simulink model "MyPowerSupply_RTW"  (Simulink 7.5)
settings: Solver=ode1  SolverMode=SingleTasking  StartTime=0.0  StopTime=inf  FixedStep=0.0002  RelTol=1e-3
PreLoadFcn:
  | vehicle = 'Car'; if ~length(which('cmcmd')), cmenv; end
  | MyPowerSupply_RTW_bus
InitFcn:
  | vehicle = 'Car'; if ~length(which('cmcmd')), cmenv; end
  | MyPowerSupply_RTW_bus
libraries: simulink x3, CarMaker4SL x3
Description:
  | CarMaker Real-Time Target (generic)
settings Model: Creator=ml  LastModifiedBy=ml
settings DebuggingCC: SolverPrmCheckMsg=none
settings HardwareCC: TargetHWDeviceType=32-bit Generic  ProdEqTarget=off
settings RTWCC: SystemTargetFile=CarMaker.tlc  TemplateMakefile=CarMaker_unix.tmf  Description=CarMaker Real-Time Target (32-bit)  ProcessScript=CarMaker_make_rtw_hook
settings CodeAppCC: MaxIdLength=63
settings STFCustomTargetCC: ModelReferenceCompliant=off  GeneratePreprocessorConditionals=Disable all  SystemTargetFile=CarMaker.tlc
settings GRTTargetCC: ModelReferenceCompliant=off  ParMdlRefBuildCompliant=off  CompOptLevelCompliant=off  MatFileLogging=off  ExtModeMexFile=noextcomm
settings CustomProperty: DataType=string  Value=..
settings EnumStrPairs: String=Car

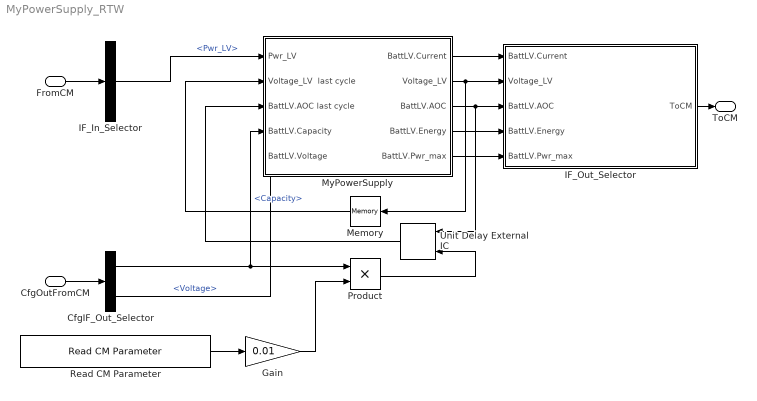
== system MyPowerSupply_RTW ==
  FromCM : Inport  UseBusObject=on
      settings: BusObject=cmPTPowerSupplyIn
  CfgOutFromCM : Inport  Port=2  UseBusObject=on
      settings: BusObject=cmPTPowerSupplyCfgOut
  CfgIF_Out_Selector : BusSelector  OutputSignals=BattLV.Capacity,BattLV.Voltage
  Gain : Gain  Gain=0.01  ParameterDataType=sfix(16)  ParameterScaling=2^0  OutDataType=sfix(16)  OutScaling=2^0
  IF_In_Selector : BusSelector  OutputSignals=Pwr_LV
  IF_Out_Selector : Subsystem
      settings: OpenFcn=cmSignalSelect('SignalSelection_CB',gcb)
      mask Type: Signal Selection
      mask Description: Signal Selection Block
  Memory : Memory
  MyPowerSupply : Subsystem
  Product : Product  OutDataType=sfix(16)  OutScaling=2^0  RndMeth=Zero
  Read CM Parameter : CarMaker4SL/Read CM Parameter  xfile=Vehicle  xkey=PowerTrain.PowerSupply.BattLV.SOC  xnout=1  xdefaults=70.0  xmuxed=on
  Unit Delay External IC : simulink/Additional Math & Discrete/Additional Discrete/Unit Delay External IC  SystemSampleTime=-1  tsamp=-1
  ToCM : Outport  UseBusObject=on
      settings: BusObject=cmPTPowerSupplyOut
  wires:
  FromCM/1 -> IF_In_Selector/1
  IF_Out_Selector/1(ToCM) -> ToCM/1
  CfgOutFromCM/1 -> CfgIF_Out_Selector/1
  Memory/1 -> MyPowerSupply/2(Voltage_LV  last cycle)
  IF_In_Selector/1 -> MyPowerSupply/1(Pwr_LV)  "<Pwr_LV>"
  MyPowerSupply/1(BattLV.Current) -> IF_Out_Selector/1(BattLV.Current)
  MyPowerSupply/2(Voltage_LV) -> Memory/1, IF_Out_Selector/2(Voltage_LV)
  MyPowerSupply/3(BattLV.AOC) -> Unit Delay External IC/1, IF_Out_Selector/3(BattLV.AOC)
  Read CM Parameter/1 -> Gain/1
  Gain/1 -> Product/2
  CfgIF_Out_Selector/1 -> Product/1, MyPowerSupply/4(BattLV.Capacity)  "<Capacity>"
  Product/1 -> Unit Delay External IC/2
  Unit Delay External IC/1 -> MyPowerSupply/3(BattLV.AOC last cycle)
  CfgIF_Out_Selector/2 -> MyPowerSupply/5(BattLV.Voltage)  "<Voltage>"
  MyPowerSupply/4(BattLV.Energy) -> IF_Out_Selector/4(BattLV.Energy)
  MyPowerSupply/5(BattLV.Pwr_max) -> IF_Out_Selector/5(BattLV.Pwr_max)

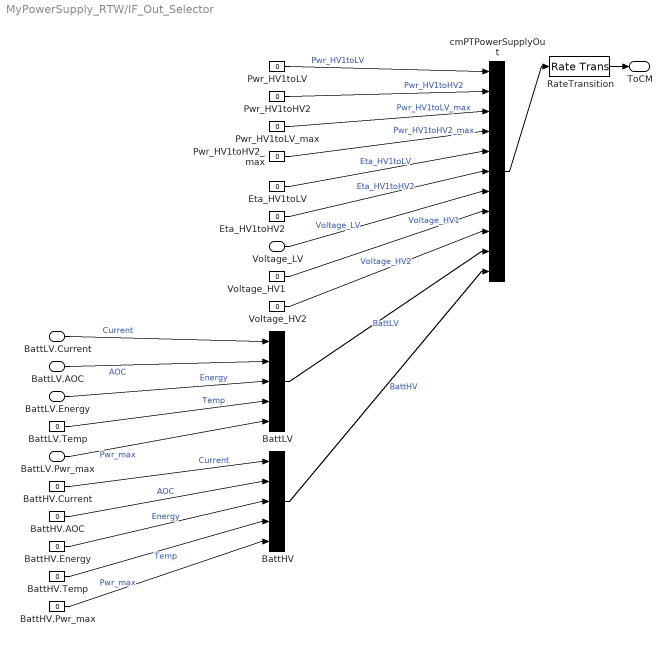
== system MyPowerSupply_RTW/IF_Out_Selector ==
  BattLV.Current : Inport
  Voltage_LV : Inport  Port=2
  BattLV.AOC : Inport  Port=3
  BattLV.Energy : Inport  Port=4
  BattLV.Pwr_max : Inport  Port=5
  BattHV : BusCreator  Inputs=5
  BattHV.AOC : Constant  Value=0
  BattHV.Current : Constant  Value=0
  BattHV.Energy : Constant  Value=0
  BattHV.Pwr_max : Constant  Value=0
  BattHV.Temp : Constant  Value=0
  BattLV : BusCreator  Inputs=5
  BattLV.Temp : Constant  Value=0
  Eta_HV1toHV2 : Constant  Value=0
  Eta_HV1toLV : Constant  Value=0
  Pwr_HV1toHV2 : Constant  Value=0
  Pwr_HV1toHV2_max : Constant  Value=0
  Pwr_HV1toLV : Constant  Value=0
  Pwr_HV1toLV_max : Constant  Value=0
  RateTransition : RateTransition  OutPortSampleTime=str2num(get_param(gcs,'FixedStep'))
  Voltage_HV1 : Constant  Value=0
  Voltage_HV2 : Constant  Value=0
  cmPTPowerSupplyOut : BusCreator  Inputs=11
  ToCM : Outport
  wires:
  RateTransition/1 -> ToCM/1
  cmPTPowerSupplyOut/1 -> RateTransition/1
  Pwr_HV1toLV/1 -> cmPTPowerSupplyOut/1  "Pwr_HV1toLV"
  Pwr_HV1toHV2/1 -> cmPTPowerSupplyOut/2  "Pwr_HV1toHV2"
  Pwr_HV1toLV_max/1 -> cmPTPowerSupplyOut/3  "Pwr_HV1toLV_max"
  Pwr_HV1toHV2_max/1 -> cmPTPowerSupplyOut/4  "Pwr_HV1toHV2_max"
  Eta_HV1toLV/1 -> cmPTPowerSupplyOut/5  "Eta_HV1toLV"
  Eta_HV1toHV2/1 -> cmPTPowerSupplyOut/6  "Eta_HV1toHV2"
  Voltage_HV1/1 -> cmPTPowerSupplyOut/8  "Voltage_HV1"
  Voltage_HV2/1 -> cmPTPowerSupplyOut/9  "Voltage_HV2"
  BattLV/1 -> cmPTPowerSupplyOut/10  "BattLV"
  BattLV.Temp/1 -> BattLV/4  "Temp"
  BattHV/1 -> cmPTPowerSupplyOut/11  "BattHV"
  BattHV.Current/1 -> BattHV/1  "Current"
  BattHV.AOC/1 -> BattHV/2  "AOC"
  BattHV.Energy/1 -> BattHV/3  "Energy"
  BattHV.Temp/1 -> BattHV/4  "Temp"
  BattHV.Pwr_max/1 -> BattHV/5  "Pwr_max"
  BattLV.Current/1 -> BattLV/1  "Current"
  Voltage_LV/1 -> cmPTPowerSupplyOut/7  "Voltage_LV"
  BattLV.AOC/1 -> BattLV/2  "AOC"
  BattLV.Energy/1 -> BattLV/3  "Energy"
  BattLV.Pwr_max/1 -> BattLV/5  "Pwr_max"

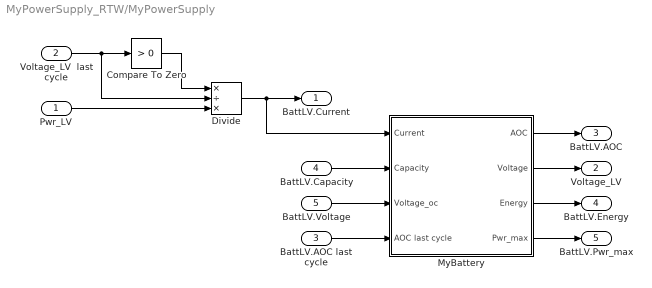
== system MyPowerSupply_RTW/MyPowerSupply ==
  Pwr_LV : Inport  OutDataType=sfix(16)  OutScaling=2^0
  Voltage_LV  last cycle : Inport  Port=2  OutDataType=sfix(16)  OutScaling=2^0
  BattLV.AOC last cycle : Inport  Port=3  OutDataType=sfix(16)  OutScaling=2^0
  BattLV.Capacity : Inport  Port=4  OutDataType=sfix(16)  OutScaling=2^0
  BattLV.Voltage : Inport  Port=5  OutDataType=sfix(16)  OutScaling=2^0
  Compare To Zero : simulink/Logic and Bit Operations/Compare To Zero  SystemSampleTime=-1  relop=>  LogicOutDataTypeMode=uint8  ZeroCross=off
  Divide : Product  Inputs=*/*  OutDataType=sfix(16)  OutScaling=2^-10
  MyBattery : Subsystem
  BattLV.Current : Outport  OutDataType=sfix(16)  OutScaling=2^0
  Voltage_LV : Outport  Port=2  OutDataType=sfix(16)  OutScaling=2^0
  BattLV.AOC : Outport  Port=3  OutDataType=sfix(16)  OutScaling=2^0
  BattLV.Energy : Outport  Port=4  OutDataType=sfix(16)  OutScaling=2^0
  BattLV.Pwr_max : Outport  Port=5  OutDataType=sfix(16)  OutScaling=2^0
  wires:
  Voltage_LV  last cycle/1 -> Compare To Zero/1, Divide/2
  Compare To Zero/1 -> Divide/1
  Pwr_LV/1 -> Divide/3
  Divide/1 -> BattLV.Current/1, MyBattery/1(Current)
  BattLV.Capacity/1 -> MyBattery/2(Capacity)
  BattLV.Voltage/1 -> MyBattery/3(Voltage_oc)
  BattLV.AOC last cycle/1 -> MyBattery/4(AOC last cycle)
  MyBattery/1(AOC) -> BattLV.AOC/1
  MyBattery/2(Voltage) -> Voltage_LV/1
  MyBattery/3(Energy) -> BattLV.Energy/1
  MyBattery/4(Pwr_max) -> BattLV.Pwr_max/1

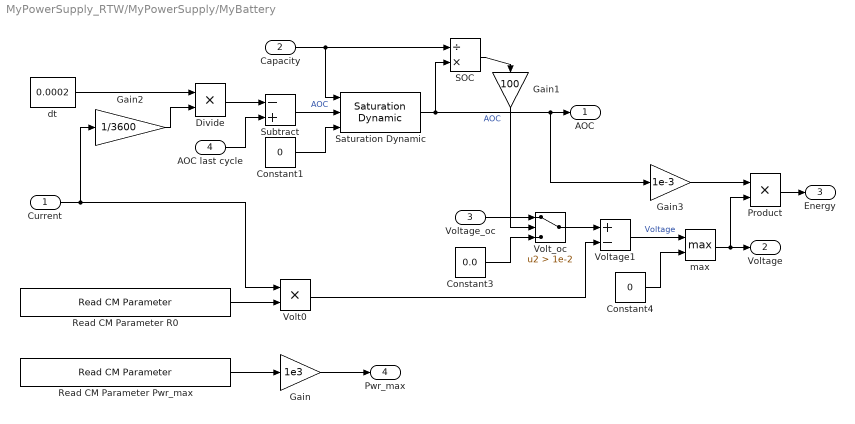
== system MyPowerSupply_RTW/MyPowerSupply/MyBattery ==
  Current : Inport  OutDataType=sfix(16)  OutScaling=2^0
  Capacity : Inport  Port=2  OutDataType=sfix(16)  OutScaling=2^0
  Voltage_oc : Inport  Port=3  OutDataType=sfix(16)  OutScaling=2^0
  AOC last cycle : Inport  Port=4  OutDataType=sfix(16)  OutScaling=2^0
  Constant1 : Constant  Value=0  OutDataType=sfix(16)  OutScaling=2^0
  Constant3 : Constant  Value=0.0  OutDataType=sfix(16)  OutScaling=2^0
  Constant4 : Constant  Value=0  OutDataType=sfix(16)  OutScaling=2^0
  Divide : Product  Inputs=**  OutDataType=sfix(16)  OutScaling=2^-10
  Gain : Gain  Gain=1e3  ParameterDataType=sfix(16)  ParameterScaling=2^0  OutDataType=sfix(16)  OutScaling=2^0
  Gain1 : Gain  Gain=100  ParameterDataType=sfix(16)  ParameterScaling=2^0  OutDataType=sfix(16)  OutScaling=2^0
  Gain2 : Gain  Gain=1/3600  ParameterDataType=sfix(16)  ParameterScaling=2^0  OutDataType=sfix(16)  OutScaling=2^0
  Gain3 : Gain  Gain=1e-3  ParameterDataType=sfix(16)  ParameterScaling=2^0  OutDataType=sfix(16)  OutScaling=2^0
  Product : Product  OutDataType=sfix(16)  OutScaling=2^0  RndMeth=Zero
  Read CM Parameter Pwr_max : CarMaker4SL/Read CM Parameter  xfile=Vehicle  xkey=PowerTrain.PowerSupply.BattLV.Pwr_max  xnout=1  xdefaults=100  xmuxed=on
  Read CM Parameter R0 : CarMaker4SL/Read CM Parameter  xfile=Vehicle  xkey=PowerTrain.PowerSupply.BattLV.R0  xnout=1  xdefaults=0.0012  xmuxed=on
  SOC : Product  Inputs=/*  OutDataType=sfix(16)  OutScaling=2^-10
  Saturation Dynamic : simulink/Discontinuities/Saturation Dynamic  SystemSampleTime=-1  OutMin=[]  OutMax=[]  OutDataTypeStr=Inherit: Same as second input  OutDataType=sfix(16)  OutScaling=2^-10  DoSatur=off
  Subtract : Sum  Inputs=-+  OutDataType=sfix(16)  OutScaling=2^-10
  Volt0 : Product  OutDataType=sfix(16)  OutScaling=2^0  RndMeth=Zero
  Volt_oc : Switch  Criteria=u2 > Threshold  Threshold=1e-2  OutDataType=sfix(16)  OutScaling=2^0
  Voltage1 : Sum  Inputs=+-  OutDataType=sfix(16)  OutScaling=2^-10
  dt : Constant  Value=0.0002  OutDataType=sfix(16)  OutScaling=2^0
  max : MinMax  Function=max  Inputs=2  OutDataType=sfix(16)  OutScaling=2^0
  AOC : Outport  OutDataType=sfix(16)  OutScaling=2^0
  Voltage : Outport  Port=2  OutDataType=sfix(16)  OutScaling=2^0
  Energy : Outport  Port=3  OutDataType=sfix(16)  OutScaling=2^0
  Pwr_max : Outport  Port=4  OutDataType=sfix(16)  OutScaling=2^0
  wires:
  Saturation Dynamic/1 -> AOC/1, Gain3/1, SOC/2  "AOC"
  Divide/1 -> Subtract/1
  dt/1 -> Divide/1
  Current/1 -> Volt0/1, Gain2/1
  Subtract/1 -> Saturation Dynamic/2  "AOC"
  Constant1/1 -> Saturation Dynamic/3
  Capacity/1 -> Saturation Dynamic/1, SOC/1
  Read CM Parameter Pwr_max/1 -> Gain/1
  SOC/1 -> Gain1/1
  Voltage_oc/1 -> Volt_oc/1
  Constant3/1 -> Volt_oc/3
  Read CM Parameter R0/1 -> Volt0/2
  Volt_oc/1 -> Voltage1/1
  Volt0/1 -> Voltage1/2
  Voltage1/1 -> max/1  "Voltage"
  Constant4/1 -> max/2
  max/1 -> Voltage/1, Product/2
  Product/1 -> Energy/1
  Gain/1 -> Pwr_max/1
  AOC last cycle/1 -> Subtract/2
  Gain2/1 -> Divide/2
  Gain3/1 -> Product/1
  Gain1/1 -> Volt_oc/2
